simulink library "Block_TestLib"  (R2017b)
settings: Solver=VariableStepAuto  StartTime=0.0  StopTime=10.0  RelTol=1e-3
settings Model: Creator=hbourbou  LastModifiedBy=hbourbou

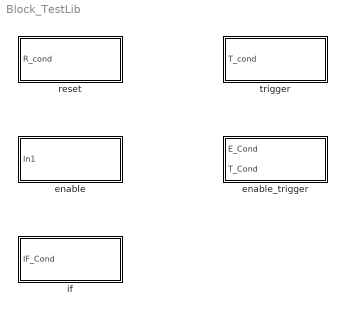
== system Block_TestLib ==
  enable : Subsystem
  enable_trigger : Subsystem
  if : Subsystem
  reset : Subsystem
  trigger : Subsystem

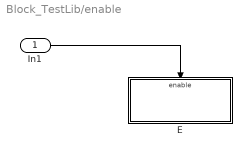
== system Block_TestLib/enable ==
  In1 : Inport  OutDataTypeStr=boolean
  E : Subsystem  TreatAsAtomicUnit=on
  wires:
  In1/1 -> E/Enable

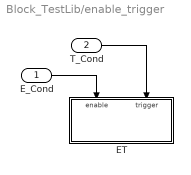
== system Block_TestLib/enable_trigger ==
  E_Cond : Inport  OutDataTypeStr=boolean
  T_Cond : Inport  Port=2  OutDataTypeStr=boolean
  ET : Subsystem  TreatAsAtomicUnit=on
  wires:
  E_Cond/1 -> ET/Enable
  T_Cond/1 -> ET/Trigger

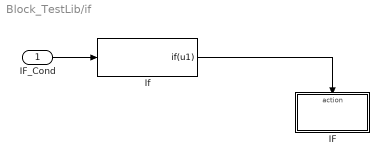
== system Block_TestLib/if ==
  IF_Cond : Inport  OutDataTypeStr=boolean
  IF : Subsystem  TreatAsAtomicUnit=on
  If : If  IfExpression=u1  ShowElse=off
  wires:
  If/1 -> IF/Action
  IF_Cond/1 -> If/1

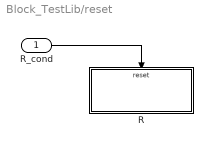
== system Block_TestLib/reset ==
  R_cond : Inport  OutDataTypeStr=boolean
  R : Subsystem  TreatAsAtomicUnit=on
  wires:
  R_cond/1 -> R/Reset

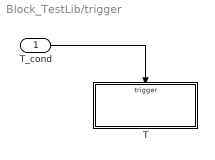
== system Block_TestLib/trigger ==
  T_cond : Inport  OutDataTypeStr=boolean
  T : Subsystem  TreatAsAtomicUnit=on
  wires:
  T_cond/1 -> T/Trigger

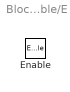
== system Block_TestLib/enable/E ==
  Enable : EnablePort

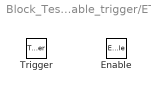
== system Block_TestLib/enable_trigger/ET ==
  Enable : EnablePort
  Trigger : TriggerPort  VariantControl=Variant

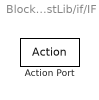
== system Block_TestLib/if/IF ==
  Action Port : ActionPort  ActionType=then

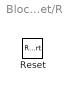
== system Block_TestLib/reset/R ==
  Reset : ResetPort  DisableCoverage=on

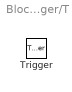
== system Block_TestLib/trigger/T ==
  Trigger : TriggerPort  VariantControl=Variant
